simulink model "modelX"  (R2020b)
settings: Solver=VariableStepAuto  StartTime=0.0  StopTime=140  RelTol=1e-3
values from neighbouring files (symbols this model uses):
  k1 = params(1)    [objectiveStaticna.m]
  k2 = params(2)    [objectiveStaticna.m]
undefined symbols (not defined in the file or in its folder): f0, J, k3, lm, psi_1, psi_2
libraries: powerlib_meascontrol x1
settings Model: Creator=64210381  LastModifiedBy=Acer

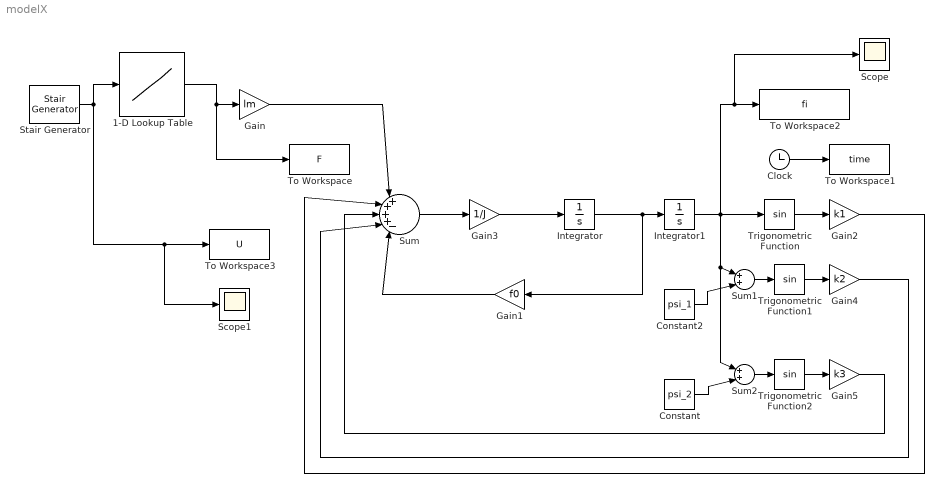
== system modelX ==
  1-D Lookup Table : Lookup_n-D  NumberOfTableDimensions=1  BreakpointsForDimension1=[0,4.6, 4.7, 5, 5.5, 6, 7, 7.5, 8, 8.5, 10]  Table=[0,0,0.10984,0.21163,0.38639,0.54977,0.83,0.9284,0.9284, 0.9284,0.9284]  InternalRulePriority=Speed  RndMeth=Simplest  InputSameDT=on
  Clock : Clock
  Constant : Constant  Value=psi_2
  Constant2 : Constant  Value=psi_1
  Gain : Gain  Gain=lm
  Gain1 : Gain  Gain=f0
  Gain2 : Gain  Gain=k1
  Gain3 : Gain  Gain=1/J
  Gain4 : Gain  Gain=k2
  Gain5 : Gain  Gain=k3
  Integrator : Integrator
  Integrator1 : Integrator
  Scope : Scope
  Scope1 : Scope
  Stair Generator : powerlib_meascontrol/Pulse & Signal Generators/Stair Generator  t=0:20:100  e=5:0.5:7.5  Ts=0
  Sum : Sum  Inputs=|++++-|
  Sum1 : Sum  Inputs=|++|
  Sum2 : Sum  Inputs=|++|
  To Workspace : ToWorkspace  VariableName=F  SampleTime=-1
  To Workspace1 : ToWorkspace  VariableName=time  SampleTime=-1
  To Workspace2 : ToWorkspace  VariableName=fi  SaveFormat=Timeseries  SampleTime=0.1
  To Workspace3 : ToWorkspace  VariableName=U  SampleTime=-1
  Trigonometric Function : Trigonometry
  Trigonometric Function1 : Trigonometry
  Trigonometric Function2 : Trigonometry
  wires:
  Trigonometric Function2/1 -> Gain5/1
  Clock/1 -> To Workspace1/1
  Integrator1/1 -> Trigonometric Function/1, To Workspace2/1, Scope/1, Sum2/1, Sum1/1
  Sum1/1 -> Trigonometric Function1/1
  Trigonometric Function1/1 -> Gain4/1
  Gain3/1 -> Integrator/1
  Stair Generator/1 -> 1-D Lookup Table/1, Scope1/1, To Workspace3/1
  Gain4/1 -> Sum/4
  Trigonometric Function/1 -> Gain2/1
  Gain2/1 -> Sum/2
  Gain/1 -> Sum/1
  Gain5/1 -> Sum/3
  Sum/1 -> Gain3/1
  Gain1/1 -> Sum/5
  Constant/1 -> Sum2/2
  Integrator/1 -> Integrator1/1, Gain1/1
  Sum2/1 -> Trigonometric Function2/1
  Constant2/1 -> Sum1/2
  1-D Lookup Table/1 -> To Workspace/1, Gain/1
